simulink model "WPC"  (R2015a)
settings: Solver=ode45  StartTime=0.0  StopTime=10.0  RelTol=1e-3
settings Model: NumberOfSteps=3  Creator=AVI  LastModifiedBy=AVI

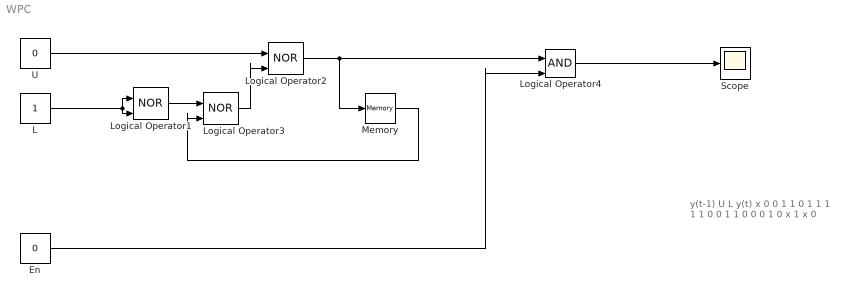
== system WPC ==
  note: y(t-1)
      | U
      | L
      | y(t)
      |
      | x
      | 0
      | 0
      | 1
      |
      | 1
      | 0
      | 1
      | 1
      |
      | 1
      | 1
      | 1
      | 0
      |
      | 0
      | 1
      | 1
      | 0
      |
      | 0
      | 0
      | 1
      | 0
      |
      | x
      | 1
      | x
      | 0
  En : Constant  Value=0  VectorParams1D=off  OutDataTypeStr=boolean
  L : Constant  VectorParams1D=off  OutDataTypeStr=boolean
  Logical Operator1 : Logic  Operator=NOR  IconShape=distinctive  AllPortsSameDT=off
  Logical Operator2 : Logic  Operator=NOR  IconShape=distinctive  AllPortsSameDT=off
  Logical Operator3 : Logic  Operator=NOR  IconShape=distinctive  AllPortsSameDT=off
  Logical Operator4 : Logic  IconShape=distinctive  AllPortsSameDT=off
  Memory : Memory  InheritSampleTime=on  LinearizeMemory=on  LinearizeAsDelay=on
  Scope : Scope
      settings: TimeRange=10  YMin=-1  YMax=2
  U : Constant  Value=0  OutDataTypeStr=boolean
  wires:
  U/1 -> Logical Operator2/1
  L/1 -> Logical Operator1/1, Logical Operator1/2
  Logical Operator3/1 -> Logical Operator2/2
  Logical Operator1/1 -> Logical Operator3/1
  Memory/1 -> Logical Operator3/2
  Logical Operator2/1 -> Logical Operator4/1, Memory/1
  Logical Operator4/1 -> Scope/1
  En/1 -> Logical Operator4/2
